simulink model "MoCo_Brake_CMcoder"  (R2019b)
settings: Solver=ode1  StartTime=0.0  StopTime=inf  FixedStep=0.001  RelTol=1e-3
PreLoadFcn:
  | vehicle = 'Car'; if ~length(which('cmself')), run ../cmenv; end
  | addpath ../../../../src/MoCo_Brake
  | run ../../../../src/MoCo_Brake/MoCo_Brake_Parameter
values from neighbouring files (symbols this model uses):
  Trq_Distrib_FL = 0.3    [BrkActuatorParameters.m]
  Trq_Distrib_FR = 0.3    [BrkActuatorParameters.m]
  Trq_Distrib_RL = 0.2    [BrkActuatorParameters.m]
  Trq_Distrib_RR = 0.2    [BrkActuatorParameters.m]
libraries: CarMaker4SL x16
Description:
  | CarMaker Plug-in Model Target
settings Model: TunableVars=Brk_SSM_Decel_Lim,Brk_SSM_Hold_Grd_Lim,Brk_SSM_Release_Grd_Lim,D_brk,K_brk,K_brk_accel_dec,K_brk_trq_dec,T_brk_accel_dec,T_brk_trq_dec,Trq_Distrib_FL,Trq_Distrib_FR,Trq_Distrib_RL,Trq_Distrib_RR,accel_to_trq,brakeBlendRange,brakeBlendStrt,brake_pres_exist_threshold,delay_brake_inc,delay_brake_inc_init,w0_brk,w0_brkinit  TunableVarsStorageClass=Auto,Auto,Auto,Auto,Auto,Auto,Auto,Auto,Auto,Auto,Auto,Auto,Auto,Auto,Auto,Auto,Auto,Auto,Auto,Auto,Auto  TunableVarsTypeQualifier=,,,,,,,,,,,,,,,,,,,,  Creator=uib55286  LastModifiedBy=uid33443
settings DataIOCC: ReturnWorkspaceOutputs=off
settings DebuggingCC: ArithmeticOperatorsInVariantConditions=warning
settings SFSimCC: CustomCodeUndefinedFunction=UseInterfaceOnly
settings RTWCC: Description=CarMaker Plug-in Model Target  SystemTargetFile=CarMaker.tlc  TemplateMakefile=CarMaker_unix-win64.tmf
settings CodeAppCC: MaxIdLength=127
settings STFCustomTargetCC: TargetLangStandard=C99 (ISO)  CombineOutputUpdateFcns=on  MultiInstanceERTCode=on  CodeInterfacePackaging=Reusable function  GenerateAllocFcn=on  SystemTargetFile=CarMaker.tlc
settings GRTTargetCC: ParMdlRefBuildCompliant=off  CompOptLevelCompliant=off  ConcurrentExecutionCompliant=off  MatFileLogging=off  MultiInstanceERTCode=on  CodeInterfacePackaging=Reusable function  CPPClassGenCompliant=off  GenerateAllocFcn=on  UseToolchainInfoCompliant=off  RTWCAPISignals=on  RTWCAPIParams=on  RTWCAPIStates=on

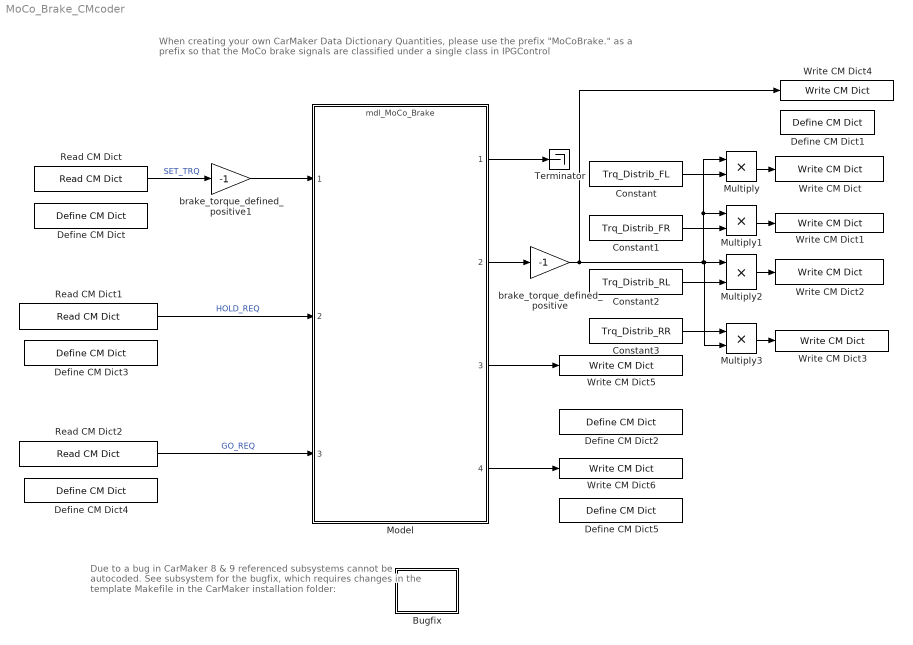
== system MoCo_Brake_CMcoder ==
  note: When creating your own CarMaker Data Dictionary Quantities, please use the prefix "MoCoBrake." as a prefix so that the MoCo brake signals are
      | classified under a single class in IPGControl
  note: Due to a bug in CarMaker 8 & 9 referenced subsystems cannot
      | be autocoded. See subsystem for the bugfix, which requires changes
      | in the template Makefile in the CarMaker installation folder:
  Bugfix : Subsystem
  Constant : Constant  Value=Trq_Distrib_FL
  Constant1 : Constant  Value=Trq_Distrib_FR
  Constant2 : Constant  Value=Trq_Distrib_RL
  Constant3 : Constant  Value=Trq_Distrib_RR
  Define CM Dict : CarMaker4SL/Define CM Dict  xname=MoCoBrake.Target_Trq  xunit=Nm  xmono=off  xtype=Double4  xdvaplace=VC  xnstates=0  xfirststate=0  xinitial=0
  Define CM Dict1 : CarMaker4SL/Define CM Dict  xname=MoCoBrake.Veh_Trq  xunit=Nm  xmono=off  xtype=Double4  xdvaplace=None  xnstates=0  xfirststate=0  xinitial=0
  Define CM Dict2 : CarMaker4SL/Define CM Dict  xname=MoCoBrake.Ssm_Status  xmono=off  xtype=Int  xdvaplace=None  xnstates=0  xfirststate=0  xinitial=0
  Define CM Dict3 : CarMaker4SL/Define CM Dict  xname=MoCoBrake.Ssm_Hold_Req  xmono=off  xtype=Int  xdvaplace=VC  xnstates=0  xfirststate=0  xinitial=0
  Define CM Dict4 : CarMaker4SL/Define CM Dict  xname=MoCoBrake.Ssm_Go_Req  xmono=off  xtype=Int  xdvaplace=VC  xnstates=0  xfirststate=0  xinitial=0
  Define CM Dict5 : CarMaker4SL/Define CM Dict  xname=MoCoBrake.Ssm_Torque  xunit=Nm  xmono=off  xtype=Int  xdvaplace=None  xnstates=0  xfirststate=0  xinitial=0
  Model : ModelReference  ModelNameDialog=mdl_MoCo_Brake.slx  SimulationMode=Normal  ModelReferenceVersion=1.3
  Multiply{,1..3} (4 alike) : Product
  Read CM Dict : CarMaker4SL/Read CM Dict  xname=MoCoBrake.Target_Trq  xsync=off
  Read CM Dict1 : CarMaker4SL/Read CM Dict  xname=MoCoBrake.Ssm_Hold_Req  xsync=off
  Read CM Dict2 : CarMaker4SL/Read CM Dict  xname=MoCoBrake.Ssm_Go_Req  xsync=off
  Terminator : Terminator
  Write CM Dict : CarMaker4SL/Write CM Dict  xname=Brake.Trq_FL_ext  xsync=off
  Write CM Dict1 : CarMaker4SL/Write CM Dict  xname=Brake.Trq_FR_ext  xsync=off
  Write CM Dict2 : CarMaker4SL/Write CM Dict  xname=Brake.Trq_RL_ext  xsync=off
  Write CM Dict3 : CarMaker4SL/Write CM Dict  xname=Brake.Trq_RR_ext  xsync=off
  Write CM Dict4 : CarMaker4SL/Write CM Dict  xname=MoCoBrake.Veh_Trq  xsync=off
  Write CM Dict5 : CarMaker4SL/Write CM Dict  xname=MoCoBrake.Ssm_Status  xsync=off
  Write CM Dict6 : CarMaker4SL/Write CM Dict  xname=MoCoBrake.Ssm_Torque  xsync=off
  brake_torque_defined_positive : Gain  Gain=-1
  brake_torque_defined_positive1 : Gain  Gain=-1
  wires:
  Read CM Dict/1 -> brake_torque_defined_positive1/1  "SET_TRQ"
  Model/1 -> Terminator/1
  Constant/1 -> Multiply/2
  Multiply/1 -> Write CM Dict/1
  Constant1/1 -> Multiply1/2
  Constant2/1 -> Multiply2/2
  Constant3/1 -> Multiply3/1
  Multiply1/1 -> Write CM Dict1/1
  Multiply3/1 -> Write CM Dict3/1
  Multiply2/1 -> Write CM Dict2/1
  Read CM Dict1/1 -> Model/2  "HOLD_REQ"
  brake_torque_defined_positive1/1 -> Model/1
  Model/2 -> brake_torque_defined_positive/1
  Model/3 -> Write CM Dict5/1
  brake_torque_defined_positive/1 -> Write CM Dict4/1, Multiply3/2, Multiply2/1, Multiply/1, Multiply1/1
  Read CM Dict2/1 -> Model/3  "GO_REQ"
  Model/4 -> Write CM Dict6/1

== system MoCo_Brake_CMcoder/Bugfix ==
  note: 1) Open the following file with an editor:
      | <IPGHOME>\carmaker\win64-8.1.1\Matlab\R2019b\CarMaker_unix-win64.tmf
      |
      | 2) Search this location (apporx line 71-74):
      | OBJS = $(MODEL).o $(patsubst rt_malloc_main.o,,$(SRCS:.c=.o))
      | ifeq ($(MODELREF_TARGET_TYPE), NONE)
      | OBJS += $(WRAPPER).o
      | endif
      |
      | 3) Move '$(MODEL).o' in the if block:
      | OBJS = $(patsubst rt_malloc_main.o,,$(SRCS:.c=.o))
      | ifeq ($(MODELREF_TARGET_TYPE), NONE)
      | OBJS += $(MODEL).o $(WRAPPER).o
      | endif
      |
      | If you want to use another CM or Matlab version, please take into account that you have to adjust the path in step 1)
